simulink model "soccer_control_generated"  (R2019b)
settings: Solver=ode3  StartTime=0.0  StopTime=inf  FixedStep=0.02  RelTol=1e-3
libraries: robotlib x39
settings Model: SimulationMode=external  Creator=vuwij  LastModifiedBy=robosoccer
settings OptimizationCC: EnhancedBackFolding=on  PassReuseOutputArgsAs=Individual arguments  ZeroExternalMemoryAtStartup=off  ZeroInternalMemoryAtStartup=off  MaxStackSize=64  OptimizeBlockOrder=speed  DifferentSizesBufferReuse=on  OptimizationCustomize=off  EfficientTunableParamExpr=on
settings DebuggingCC: ParameterTunabilityLossMsg=error
settings HardwareCC: ProdBitPerPointer=32  ProdBitPerSizeT=32  ProdBitPerPtrDiffT=32  ProdLargestAtomicFloat=None  ProdIntDivRoundTo=Undefined  ProdEndianess=Unspecified  ProdWordSize=32  ProdHWDeviceType=Generic->Unspecified (assume 32-bit Generic)
settings SFSimCC: MATLABDynamicMemAlloc=off
settings RTWCC: SystemTargetFile=ert.tlc  HardwareBoard=Robot Operating System (ROS)  TLCOptions="-aInlineSetEventsForThisBaseRateFcn=TLC_FALSE -aSuppressMultiTaskScheduler=TLC_FALSE  -aRateBasedStepFcn=0"  TemplateMakefile=ert_default_tmf  GenerateReport=on  Toolchain=Catkin  IncludeHyperlinkInReport=on  LaunchReport=on  TargetLang=C++  GenerateTraceInfo=on  GenerateTraceReport=on  GenerateTraceReportSl=on  GenerateTraceReportSf=on  GenerateTraceReportEml=on
settings CodeAppCC: ForceParamTrailComments=on  IgnoreCustomStorageClasses=off  OperatorAnnotations=on  SimulinkDataObjDesc=on  SFDataObjDesc=on  InsertBlockDesc=on
settings ERTTargetCC: ExtMode=on  ExtModeMexArgs='' 0 17725

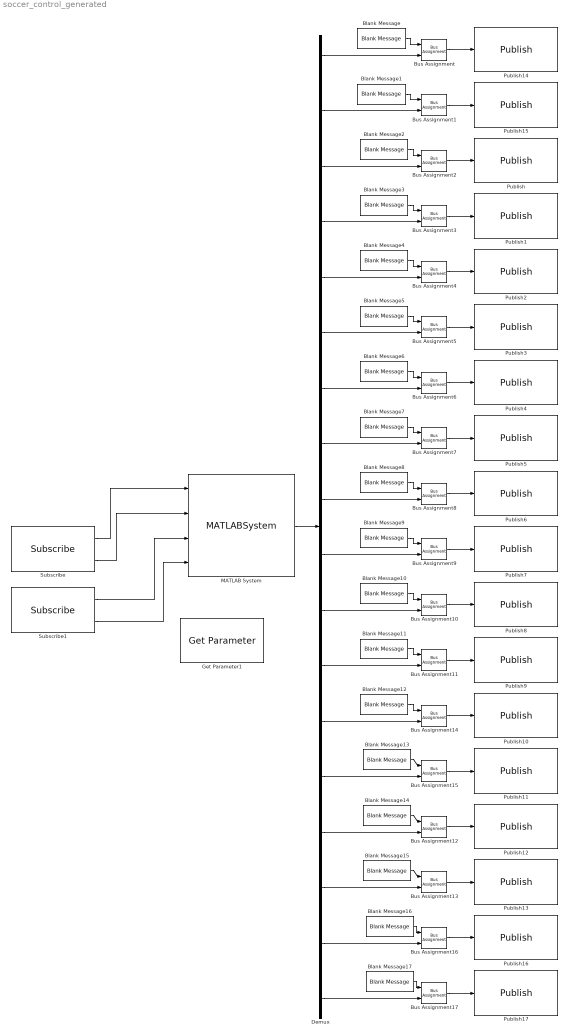
== system soccer_control_generated ==
  Blank Message{,1..17} (18 alike) : robotlib/Blank Message  messageClass=Message  entityType=std_msgs/Float64  messageType=std_msgs/Float64  SampleTime=inf
      settings: SourceProductName=ROS Toolbox
  Bus Assignment{,1..17} (18 alike) : BusAssignment  AssignedSignals=Data
  Demux : Demux  Outputs=18
  Get Parameter1 : robotlib/Get Parameter  ParameterSource=Select from ROS network  ParameterName=/my_param  ParameterType=double  ParameterMaxArrayLength=16  ParameterInitialValue=0.0  SampleTime=-1  ShowErrorCodeOutput=on  ModelName=soccer_control_generated  BlockId=ParamGet_soccer_control_generated_74
      settings: SourceProductName=ROS Toolbox  SourceProductBaseCode=RR
  MATLAB System : MATLABSystem  System=Robot.soccer_system  SimulateUsing=Code generation
      mask Type: Robot.soccer_system
      mask Display:
      | disp('soccer_system');
      | port_label('input',1,'has_new_goal');
      | port_label('input',2,'new_goal');
      | port_label('input',3,'~');
      | port_label('input',4,'new_pose');
      | port_label('output',1,'configuration');
  Publish : robotlib/Publish  topicSource=Select from ROS network  topic=/robot1/left_arm_motor_0/command  messageType=std_msgs/Float64  messageQueueLength=1
      settings: SourceProductName=ROS Toolbox
  Publish1 : robotlib/Publish  topicSource=Select from ROS network  topic=/left_arm_motor_1/command  messageType=std_msgs/Float64  messageQueueLength=1
      settings: SourceProductName=ROS Toolbox
  Publish10 : robotlib/Publish  topicSource=Select from ROS network  topic=/right_leg_motor_0/command  messageType=std_msgs/Float64  messageQueueLength=1
      settings: SourceProductName=ROS Toolbox
  Publish11 : robotlib/Publish  topicSource=Select from ROS network  topic=/right_leg_motor_1/command  messageType=std_msgs/Float64  messageQueueLength=1
      settings: SourceProductName=ROS Toolbox
  Publish12 : robotlib/Publish  topicSource=Select from ROS network  topic=/right_leg_motor_2/command  messageType=std_msgs/Float64  messageQueueLength=1
      settings: SourceProductName=ROS Toolbox
  Publish13 : robotlib/Publish  topicSource=Select from ROS network  topic=/right_leg_motor_3/command  messageType=std_msgs/Float64  messageQueueLength=1
      settings: SourceProductName=ROS Toolbox
  Publish14 : robotlib/Publish  topicSource=Select from ROS network  topic=/robot1/head_motor_0/command  messageType=std_msgs/Float64  messageQueueLength=1
      settings: SourceProductName=ROS Toolbox
  Publish15 : robotlib/Publish  topicSource=Select from ROS network  topic=/robot1/head_motor_1/command  messageType=std_msgs/Float64  messageQueueLength=1
      settings: SourceProductName=ROS Toolbox
  Publish16 : robotlib/Publish  topicSource=Select from ROS network  topic=/right_leg_motor_4/command  messageType=std_msgs/Float64  messageQueueLength=1
      settings: SourceProductName=ROS Toolbox
  Publish17 : robotlib/Publish  topicSource=Select from ROS network  topic=/right_leg_motor_5/command  messageType=std_msgs/Float64  messageQueueLength=1
      settings: SourceProductName=ROS Toolbox
  Publish2 : robotlib/Publish  topicSource=Select from ROS network  topic=/left_leg_motor_0/command  messageType=std_msgs/Float64  messageQueueLength=1
      settings: SourceProductName=ROS Toolbox
  Publish3 : robotlib/Publish  topicSource=Select from ROS network  topic=/left_leg_motor_1/command  messageType=std_msgs/Float64  messageQueueLength=1
      settings: SourceProductName=ROS Toolbox
  Publish4 : robotlib/Publish  topicSource=Select from ROS network  topic=/left_leg_motor_2/command  messageType=std_msgs/Float64  messageQueueLength=1
      settings: SourceProductName=ROS Toolbox
  Publish5 : robotlib/Publish  topicSource=Select from ROS network  topic=/left_leg_motor_3/command  messageType=std_msgs/Float64  messageQueueLength=1
      settings: SourceProductName=ROS Toolbox
  Publish6 : robotlib/Publish  topicSource=Select from ROS network  topic=/left_leg_motor_4/command  messageType=std_msgs/Float64  messageQueueLength=1
      settings: SourceProductName=ROS Toolbox
  Publish7 : robotlib/Publish  topicSource=Select from ROS network  topic=/left_leg_motor_5/command  messageType=std_msgs/Float64  messageQueueLength=1
      settings: SourceProductName=ROS Toolbox
  Publish8 : robotlib/Publish  topicSource=Select from ROS network  topic=/right_arm_motor_0/command  messageType=std_msgs/Float64  messageQueueLength=1
      settings: SourceProductName=ROS Toolbox
  Publish9 : robotlib/Publish  topicSource=Select from ROS network  topic=/right_arm_motor_1/command  messageType=std_msgs/Float64  messageQueueLength=1
      settings: SourceProductName=ROS Toolbox
  Subscribe : robotlib/Subscribe  topicSource=Specify your own  topic=/robot1/goal  messageType=geometry_msgs/Pose2D  sampleTime=-1  messageQueueLength=1
      settings: SourceProductName=ROS Toolbox
  Subscribe1 : robotlib/Subscribe  topicSource=Select from ROS network  topic=/robot1/amcl_pose  messageType=geometry_msgs/PoseWithCovarianceStamped  sampleTime=-1  messageQueueLength=1
      settings: SourceProductName=ROS Toolbox
  wires:
  Demux/18 -> Bus Assignment17/2
  Demux/17 -> Bus Assignment16/2
  Demux/16 -> Bus Assignment13/2
  Demux/15 -> Bus Assignment12/2
  Demux/14 -> Bus Assignment15/2
  Demux/13 -> Bus Assignment14/2
  Demux/12 -> Bus Assignment11/2
  Demux/11 -> Bus Assignment10/2
  Demux/10 -> Bus Assignment9/2
  Demux/9 -> Bus Assignment8/2
  Demux/8 -> Bus Assignment7/2
  Demux/7 -> Bus Assignment6/2
  Demux/6 -> Bus Assignment5/2
  Demux/5 -> Bus Assignment4/2
  Demux/4 -> Bus Assignment3/2
  Demux/3 -> Bus Assignment2/2
  Demux/2 -> Bus Assignment1/2
  Bus Assignment/1 -> Publish14/1
  MATLAB System/1 -> Demux/1
  Blank Message/1 -> Bus Assignment/1
  Demux/1 -> Bus Assignment/2
  Bus Assignment1/1 -> Publish15/1
  Bus Assignment2/1 -> Publish/1
  Bus Assignment3/1 -> Publish1/1
  Bus Assignment4/1 -> Publish2/1
  Bus Assignment5/1 -> Publish3/1
  Bus Assignment6/1 -> Publish4/1
  Bus Assignment7/1 -> Publish5/1
  Bus Assignment8/1 -> Publish6/1
  Bus Assignment9/1 -> Publish7/1
  Bus Assignment10/1 -> Publish8/1
  Bus Assignment11/1 -> Publish9/1
  Bus Assignment14/1 -> Publish10/1
  Bus Assignment15/1 -> Publish11/1
  Bus Assignment12/1 -> Publish12/1
  Bus Assignment13/1 -> Publish13/1
  Bus Assignment16/1 -> Publish16/1
  Bus Assignment17/1 -> Publish17/1
  Blank Message1/1 -> Bus Assignment1/1
  Blank Message2/1 -> Bus Assignment2/1
  Blank Message3/1 -> Bus Assignment3/1
  Blank Message4/1 -> Bus Assignment4/1
  Blank Message5/1 -> Bus Assignment5/1
  Blank Message6/1 -> Bus Assignment6/1
  Blank Message7/1 -> Bus Assignment7/1
  Blank Message8/1 -> Bus Assignment8/1
  Blank Message9/1 -> Bus Assignment9/1
  Blank Message10/1 -> Bus Assignment10/1
  Blank Message11/1 -> Bus Assignment11/1
  Blank Message12/1 -> Bus Assignment14/1
  Blank Message13/1 -> Bus Assignment15/1
  Blank Message14/1 -> Bus Assignment12/1
  Blank Message15/1 -> Bus Assignment13/1
  Blank Message16/1 -> Bus Assignment16/1
  Blank Message17/1 -> Bus Assignment17/1
  Subscribe/1 -> MATLAB System/1
  Subscribe/2 -> MATLAB System/2
  Subscribe1/1 -> MATLAB System/3
  Subscribe1/2 -> MATLAB System/4
